simulink model "RLCsubsystem"  (Simulink 7.1)
settings: Solver=ode45  StartTime=0.0  StopTime=.03  RelTol=1e-3
undefined symbols (not defined in the file): C, L, R, V
settings Model: Creator=Smrit  LastModifiedBy=Smrit

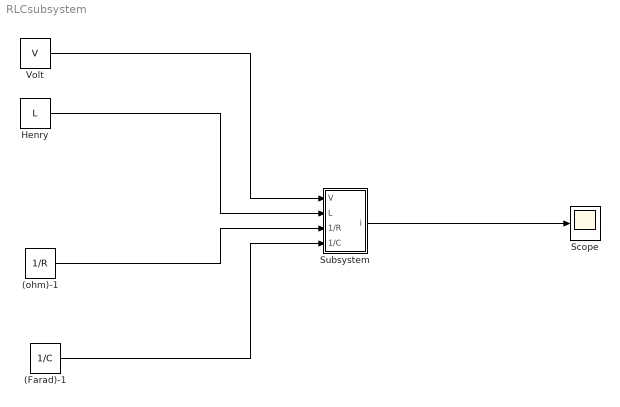
== system RLCsubsystem ==
  (Farad)-1 : Constant  Value=1/C  OutDataType=sfix(16)  OutScaling=2^0
  (ohm)-1 : Constant  Value=1/R  OutDataType=sfix(16)  OutScaling=2^0
  Henry : Constant  Value=L  OutDataType=sfix(16)  OutScaling=2^0
  Scope : Scope
  Subsystem : Subsystem
  Volt : Constant  Value=V  OutDataType=sfix(16)  OutScaling=2^0
  wires:
  Henry/1 -> Subsystem/2(L)
  Volt/1 -> Subsystem/1(V)
  (Farad)-1/1 -> Subsystem/4(1/C)
  (ohm)-1/1 -> Subsystem/3(1/R)
  Subsystem/1(i) -> Scope/1

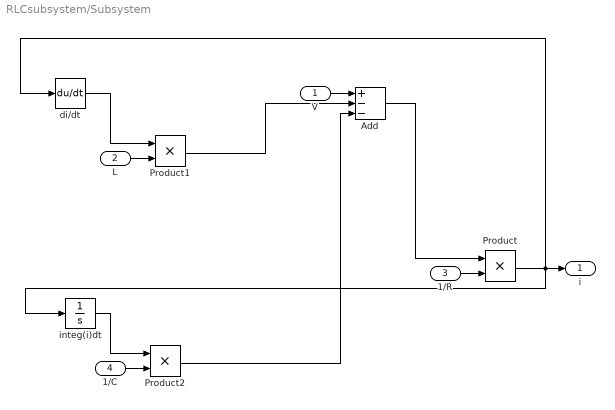
== system RLCsubsystem/Subsystem ==
  V : Inport
  L : Inport  Port=2
  1/R : Inport  Port=3
  1/C : Inport  Port=4
  Add : Sum  Inputs=+--  OutDataType=sfix(16)  OutScaling=2^-10
  Product : Product  OutDataType=sfix(16)  OutScaling=2^0  RndMeth=Zero
  Product1 : Product  OutDataType=sfix(16)  OutScaling=2^0  RndMeth=Zero
  Product2 : Product  OutDataType=sfix(16)  OutScaling=2^0  RndMeth=Zero
  di/dt : Derivative
  integ(i)dt : Integrator
  i : Outport
  wires:
  di/dt/1 -> Product1/1
  Product1/1 -> Add/2
  integ(i)dt/1 -> Product2/1
  Product2/1 -> Add/3
  Add/1 -> Product/1
  Product/1 -> di/dt/1, integ(i)dt/1, i/1
  V/1 -> Add/1
  L/1 -> Product1/2
  1/R/1 -> Product/2
  1/C/1 -> Product2/2
